simulink model "manipulatorNLMPC"  (R2023a)
settings: Solver=VariableStepAuto  StartTime=0.0  StopTime=10  RelTol=1e-3
values from neighbouring files (symbols this model uses):
  x0 = [-2;-1;1;1]    [ControlOfRobotManipulatorUsingPassivityBasedNonlinearMPC1.m]
libraries: mpclib x1
settings Model: Creator=The MathWorks, Inc.  LastModifiedBy=The MathWorks, Inc.
settings SolverCC: MaxZcPerStep=1
settings OptimizationCC: ReuseModelBlockBuffer=off
settings DebuggingCC: UnconnectedInputMsg=warning  UnconnectedOutputMsg=warning  UnconnectedLineMsg=warning
settings ModelReferenceCC: EnableRefExpFcnMdlSchedulingChecks=on
settings RTWCC: DLArmComputeVersion=19.05

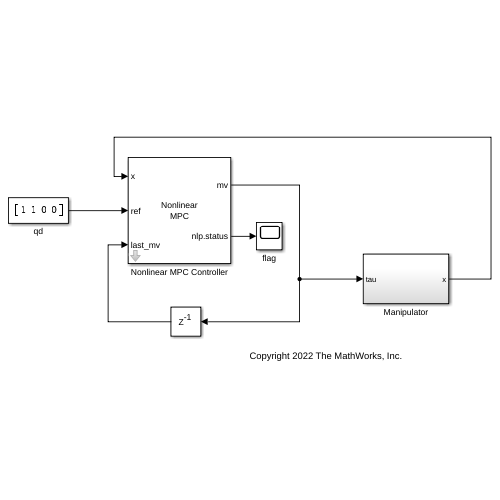
[thumbnail: Simulink's stored preview of the top-level diagram]
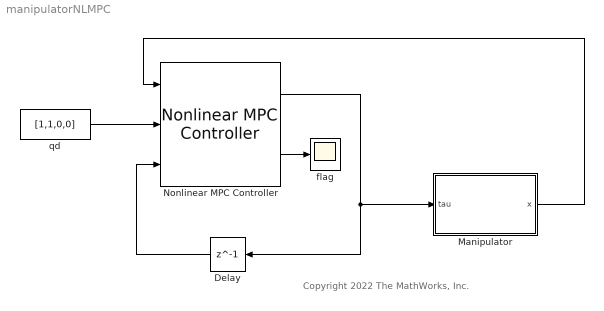
== system manipulatorNLMPC ==
  note: Copyright 2022 The MathWorks, Inc.
  Delay : Delay  DelayLength=1  InitialCondition=0
  Manipulator : Subsystem
  Nonlinear MPC Controller : mpclib/Nonlinear MPC Controller  nlmpcobj=nlobj  UseObjectTs=on  UseMEX=off  md_enabled=off  mvtarget_enabled=off  param_enabled=off  cost_enabled=off  mvseq_enabled=off  stateseq_enabled=off  ovseq_enabled=off  slack_enabled=off  status_enabled=on  ov_min=off  ov_max=off  mv_min=off  mv_max=off  mvrate_min=off  mvrate_max=off  state_min=off  state_max=off  ov_weight=off  mv_weight=off  mvrate_weight=off  ecr_weight=off  nlp_initialize=off
  flag : Scope
  qd : Constant  Value=[1,1,0,0]  VectorParams1D=off
  wires:
  Nonlinear MPC Controller/1 -> Delay/1, Manipulator/1(tau)
  Delay/1 -> Nonlinear MPC Controller/3
  Manipulator/1(x) -> Nonlinear MPC Controller/1
  Nonlinear MPC Controller/2 -> flag/1
  qd/1 -> Nonlinear MPC Controller/2

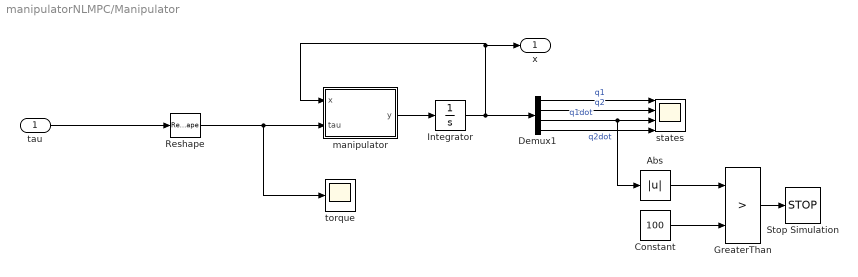
== system manipulatorNLMPC/Manipulator ==
  tau : Inport
  Abs : Abs  SaturateOnIntegerOverflow=off
  Constant : Constant  Value=100
  Demux1 : Demux
  GreaterThan : RelationalOperator  Operator=>  OutDataTypeStr=boolean  RndMeth=Simplest  InputSameDT=off
  Integrator : Integrator  InitialCondition=x0
  Reshape : Reshape  OutputDimensionality=Customize  OutputDimensions=[2,1]
  Stop Simulation : Stop
  manipulator : MATLAB Function  TreatAsAtomicUnit=on
  states : Scope  NumInputPorts=4
  torque : Scope
  x : Outport
  wires:
  manipulator/1(y) -> Integrator/1
  tau/1 -> Reshape/1
  Reshape/1 -> torque/1, manipulator/2(tau)
  Demux1/3 -> Abs/1, states/3  "q1dot"
  Demux1/2 -> states/2  "q2"
  Demux1/1 -> states/1  "q1"
  Demux1/4 -> states/4  "q2dot"
  Integrator/1 -> Demux1/1, manipulator/1(x), x/1
  GreaterThan/1 -> Stop Simulation/1
  Constant/1 -> GreaterThan/2
  Abs/1 -> GreaterThan/1

== matlab function manipulatorNLMPC/Manipulator/manipulator ==
  data: x input; tau input; y output
function y = fcn(x, tau)
y = manipulatorStateFcn(x,tau);
